simulink model "labTHREEtaskONE"  (R2023b)
settings: Solver=VariableStepAuto  StartTime=0.0  StopTime=10.0  RelTol=1e-3
libraries: simulink x2
settings Model: Creator=omarf  LastModifiedBy=omarf

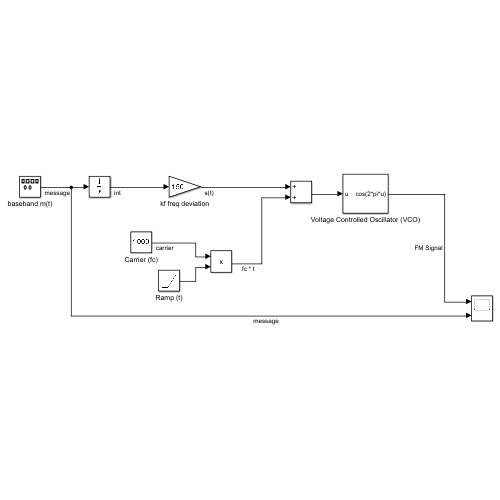
[thumbnail: Simulink's stored preview of the top-level diagram]
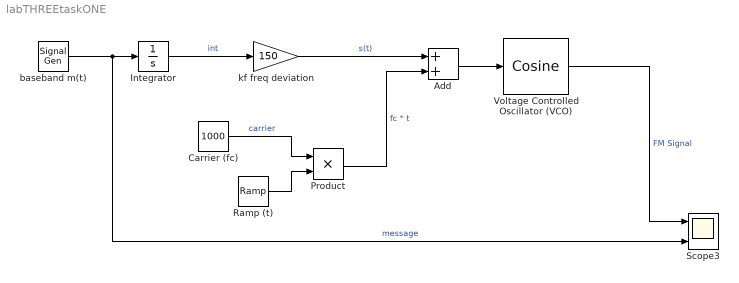
== system labTHREEtaskONE ==
  Add : Sum
  Carrier (fc) : Constant  Value=1000
  Integrator : Integrator
  Product : Product
  Ramp (t) : simulink/Sources/Ramp  slope=1  start=0  InitialOutput=0
  Scope3 : Scope  NumInputPorts=2
  Voltage Controlled Oscillator (VCO) : simulink/Lookup Tables/Cosine  Formula=cos(2*pi*u)  NumDataPoints=(2^5)+1  OutputWordLength=16  InternalRulePriority=Speed
  baseband m(t) : SignalGenerator  Amplitude=2  Frequency=100
  kf freq deviation : Gain  Gain=150
  wires:
  Carrier (fc)/1 -> Product/1  "carrier"
  baseband m(t)/1 -> Scope3/2, Integrator/1  "message"
  Integrator/1 -> kf freq deviation/1  "int"
  kf freq deviation/1 -> Add/1  "s(t)"
  Ramp (t)/1 -> Product/2
  Product/1 -> Add/2  "fc * t"
  Add/1 -> Voltage Controlled Oscillator (VCO)/1
  Voltage Controlled Oscillator (VCO)/1 -> Scope3/1  "FM Signal"
